simulink model "ballOnly_ident"  (R2017a)
settings: Solver=FixedStepAuto  StartTime=0.0  StopTime=30  FixedStep=1/50  RelTol=1e-3
undefined symbols (not defined in the file or in its folder): prms
libraries: raspi_library x2
settings Model: SimulationMode=external  ExtModeTrigDuration=10000  Creator=The MathWorks Inc.  LastModifiedBy=marti
settings SolverCC: PositivePriorityOrder=on
settings DataIOCC: LimitDataPoints=on  SaveFormat=Array
settings OptimizationCC: BlockReduction=off  BooleanDataType=off  DefaultUnderspecifiedDataType=single  LifeSpan=inf  MaxStackSize=64
settings DebuggingCC: SaveWithParameterizedLinksMsg=none  UnderspecifiedInitializationDetection=Classic  MergeDetectMultiDrivingBlocksExec=none  SignalResolutionControl=TryResolveAllWithWarning  ParameterTunabilityLossMsg=error  SFUnexpectedBacktrackingDiag=warning  SFNoUnconditionalDefaultTransitionDiag=warning  SFExecutionAtInitializationDiag=none
settings HardwareCC: ProdBitPerPointer=32  ProdBitPerSizeT=32  ProdBitPerPtrDiffT=32  ProdLargestAtomicInteger=Long  ProdLargestAtomicFloat=Double  ProdWordSize=32  ProdHWDeviceType=ARM Compatible->ARM Cortex
settings ModelReferenceCC: PropagateSignalLabelsOutOfModel=off
settings SFSimCC: MATLABDynamicMemAlloc=off
settings RTWCC: SystemTargetFile=ert.tlc  HardwareBoard=Raspberry Pi  TLCOptions=-aInlineSetEventsForThisBaseRateFcn=TLC_FALSE -aSuppressMultiTaskScheduler=TLC_FALSE -aRateBasedStepFcn=0  TemplateMakefile=ert_default_tmf  Description=Embedded Coder  GenerateReport=on  RTWVerbose=off  Toolchain=GNU GCC Raspberry Pi  BuildConfiguration=Specify  IncludeHyperlinkInReport=on  GenerateTraceInfo=on  GenerateTraceReport=on  GenerateTraceReportSl=on  GenerateTraceReportSf=on  GenerateTraceReportEml=on
settings CodeAppCC: ForceParamTrailComments=on  IgnoreCustomStorageClasses=off  OperatorAnnotations=on  SimulinkDataObjDesc=on  SFDataObjDesc=on  MATLABFcnDesc=on  MangleLength=10  InsertBlockDesc=on  MATLABSourceComments=on
settings ERTTargetCC: MultiwordLength=2048  SupportVariableSizeSignals=on
settings ConfigComp: CovMetricSettings=dw  CovHtmlReporting=on  CovSaveCumulativeToWorkspaceVar=on  CovSaveSingleToWorkspaceVar=on  CovExternalEMLEnable=off  CovSFcnEnable=off

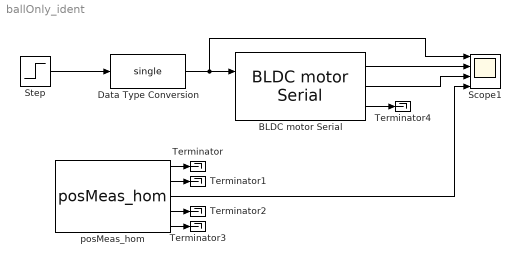
== system ballOnly_ident ==
  BLDC motor Serial : raspi_library/BLDC motor Serial  sampleTime=prms.Ts
  Data Type Conversion : DataTypeConversion  OutDataTypeStr=single
  Scope1 : Scope  NumInputPorts=4
  Step : Step  Time=0  After=0  SampleTime=prms.Ts
  Terminator{,1..4} (5 alike) : Terminator
  posMeas_hom : raspi_library/posMeas_hom  H=H  sampleTime=prms.Ts
  wires:
  Step/1 -> Data Type Conversion/1
  Data Type Conversion/1 -> Scope1/1, BLDC motor Serial/1
  posMeas_hom/1 -> Terminator/1
  posMeas_hom/2 -> Terminator1/1
  posMeas_hom/4 -> Terminator2/1
  posMeas_hom/5 -> Terminator3/1
  BLDC motor Serial/1 -> Scope1/2
  BLDC motor Serial/2 -> Scope1/3
  posMeas_hom/3 -> Scope1/4
  BLDC motor Serial/3 -> Terminator4/1
